simulink model "sampling"  (R2016b)
settings: Solver=VariableStepAuto  StartTime=0.0  StopTime=1000  MaxStep=0.001  RelTol=1e-3
libraries: dsparch4 x1
settings Model: Creator=fhs42090  LastModifiedBy=fhs42090

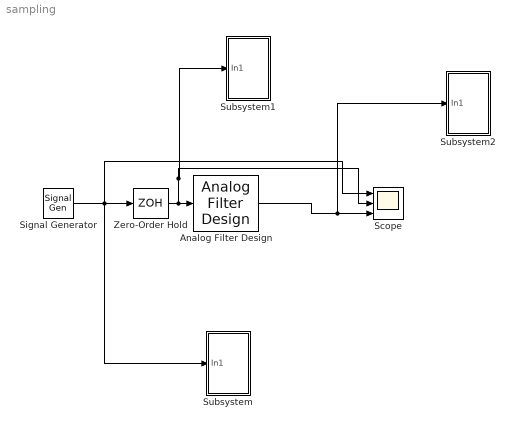
== system sampling ==
  Analog Filter Design : dsparch4/Analog Filter Design  method=Butterworth  filttype=Lowpass  N=20  Wlo=2.3*2*pi  Whi=80  Rp=2  Rs=40
  Scope : Scope  NumInputPorts=3
  Signal Generator : SignalGenerator
  Subsystem : Subsystem
  Subsystem1 : Subsystem
  Subsystem2 : Subsystem
  Zero-Order Hold : ZeroOrderHold  SampleTime=1/5
  wires:
  Zero-Order Hold/1 -> Subsystem1/1(In1), Scope/2, Analog Filter Design/1
  Analog Filter Design/1 -> Subsystem2/1(In1), Scope/3
  Signal Generator/1 -> Subsystem/1(In1), Scope/1, Zero-Order Hold/1

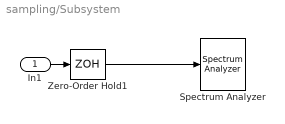
== system sampling/Subsystem ==
  In1 : Inport
  Spectrum Analyzer : SpectrumAnalyzer
  Zero-Order Hold1 : ZeroOrderHold  SampleTime=1/20
  wires:
  Zero-Order Hold1/1 -> Spectrum Analyzer/1
  In1/1 -> Zero-Order Hold1/1

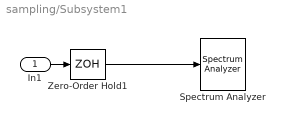
== system sampling/Subsystem1 ==
  In1 : Inport
  Spectrum Analyzer : SpectrumAnalyzer
  Zero-Order Hold1 : ZeroOrderHold  SampleTime=1/20
  wires:
  In1/1 -> Zero-Order Hold1/1
  Zero-Order Hold1/1 -> Spectrum Analyzer/1

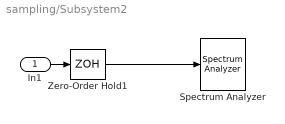
== system sampling/Subsystem2 ==
  In1 : Inport
  Spectrum Analyzer : SpectrumAnalyzer
  Zero-Order Hold1 : ZeroOrderHold  SampleTime=1/20
  wires:
  Zero-Order Hold1/1 -> Spectrum Analyzer/1
  In1/1 -> Zero-Order Hold1/1
